simulink model "modelo_SI"  (R2019b)
settings: Solver=VariableStepAuto  StartTime=0.0  StopTime=300  RelTol=1e-3
settings Model: Creator=lucia  LastModifiedBy=lucia

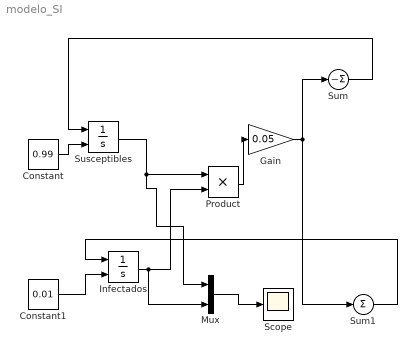
== system modelo_SI ==
  Constant : Constant  Value=0.99
  Constant1 : Constant  Value=0.01
  Gain : Gain  Gain=0.05
  Infectados : Integrator  InitialConditionSource=external
  Mux : Mux  Inputs=2
  Product : Product
  Scope : Scope
  Sum : Sum  Inputs=-
  Sum1 : Sum  Inputs=+
  Susceptibles : Integrator  InitialConditionSource=external
  wires:
  Constant/1 -> Susceptibles/2
  Infectados/1 -> Product/2, Mux/2
  Susceptibles/1 -> Mux/1, Product/1
  Product/1 -> Gain/1
  Gain/1 -> Sum1/1, Sum/1
  Sum/1 -> Susceptibles/1
  Constant1/1 -> Infectados/2
  Sum1/1 -> Infectados/1
  Mux/1 -> Scope/1
